simulink model "untitled"  (R2013a)
settings: Solver=ode45  StartTime=0.0  StopTime=10.0  RelTol=1e-3
undefined symbols (not defined in the file or in its folder): alpha
libraries: dspxfrm3 x2, dspvision x1
settings Model: Creator=hp  LastModifiedBy=hp

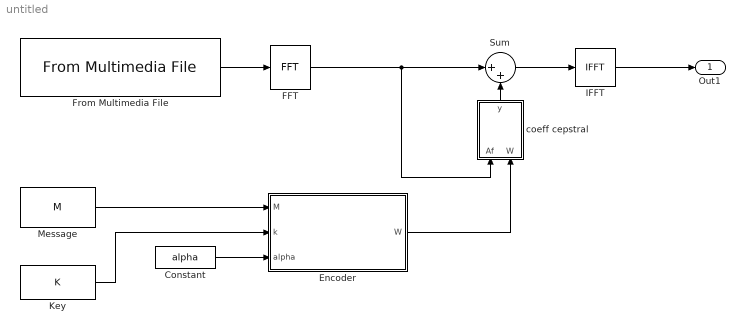
== system untitled ==
  Constant : Constant  Value=alpha
  Encoder : MATLAB Function  TreatAsAtomicUnit=on
  FFT : dspxfrm3/FFT  CompMethod=Table lookup  TableOpt=NEW  TableOptActive=Speed  BitRevOrder=off  InheritFFTLength=on  FFTLength=64  RowConvenienceOn=on  FFTImplementation=Auto  SkipNorm=off  firstCoeffDataTypeStr=Inherit: Same word length as input  firstCoeffLastDataTypeStr=Inherit: Same word length as input  outputMin=[]  outputMax=[]  roundingMode=Floor  overflowMode=off
  From Multimedia File : dspvision/From Multimedia File  inputFilename=audio1.wav  loop=on  numPlays=inf  outputStreams=Audio only  videoDataType=single  audioDataType=int16  inheritSampleTime=on  userDefinedSampleTime=1/30  noAudioOutput=off  isIntensityVideo=off  fourcc=RGB  colorVideoFormat=One multidimensional signal  outputEOF=off  dataOrg=Column-major  audioFrameSize=1024  computeAudioFrameSize=off  outSamplingMode=Sample based
  IFFT : dspxfrm3/IFFT  CompMethod=Table lookup  TableOpt=NEW  TableOptActive=Speed  BitRevOrder=off  cs_in=off  SkipNorm=on  InheritFFTLength=on  FFTLength=64  mode=Complex  outSamplingMode=Sample based  RowConvenienceOn=on  FFTImplementation=Auto  firstCoeffDataTypeStr=Inherit: Same word length as input  firstCoeffLastDataTypeStr=Inherit: Same word length as input  outputMin=[]  outputMax=[]  roundingMode=Floor  overflowMode=off
  Key : FromWorkspace  VariableName=K  SampleTime=0
  Message : FromWorkspace  VariableName=M  SampleTime=0
  Sum : Sum  Inputs=|++
  coeff cepstral : MATLAB Function  TreatAsAtomicUnit=on
  Out1 : Outport
  wires:
  From Multimedia File/1 -> FFT/1
  Message/1 -> Encoder/1(M)
  FFT/1 -> coeff cepstral/1(Af), Sum/1
  Constant/1 -> Encoder/3(alpha)
  Key/1 -> Encoder/2(k)
  Encoder/1(W) -> coeff cepstral/2(W)
  Sum/1 -> IFFT/1
  coeff cepstral/1(y) -> Sum/2
  IFFT/1 -> Out1/1

== matlab function untitled/coeff cepstral ==
  data: Af input; y output; W input
function y = fcn(Af,W)
%#codegen

y = u;

== matlab function untitled/Encoder ==
  data: M input; W output; k input; alpha input
function W = fcn(M,k,alpha)
%#codegen

W = u;
